simulink model "Simulink_Blocks"  (R2017b)
settings: Solver=FixedStepAuto  StartTime=0.0  StopTime=10.0  FixedStep=0.1  RelTol=1e-3  EnableMultiTasking=on
settings Model: Creator=yue  LastModifiedBy=changgang
settings OptimizationCC: LifeSpan=inf
settings DebuggingCC: SFUnexpectedBacktrackingDiag=warning  SFNoUnconditionalDefaultTransitionDiag=warning  SFExecutionAtInitializationDiag=none
settings CodeAppCC: StateflowObjectComments=on
settings GRTTargetCC: TargetLangStandard=C89/C90 (ANSI)  GeneratePreprocessorConditionals=Disable all
settings ConfigComp: CovMetricSettings=dw  CovHtmlReporting=on  CovSaveCumulativeToWorkspaceVar=on  CovSaveSingleToWorkspaceVar=on  CovExternalEMLEnable=off

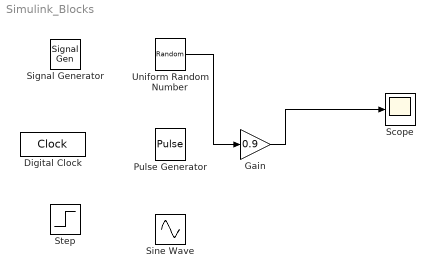
== system Simulink_Blocks ==
  Digital Clock : DigitalClock
  Gain : Gain  Gain=0.9
  Pulse Generator : DiscretePulseGenerator  PulseType=Time based  PulseWidth=70
  Scope : Scope
  Signal Generator : SignalGenerator  Units=rad/sec
  Sine Wave : Sin  SampleTime=0
  Step : Step  SampleTime=0
  Uniform Random Number : UniformRandomNumber  Minimum=-2  SampleTime=0.3
  wires:
  Gain/1 -> Scope/1
  Uniform Random Number/1 -> Gain/1
